simulink subsystem "Compute_LVLH_State"  (R2023a)
settings: Solver=VariableStepAuto  StartTime=0.0  StopTime=10.0  RelTol=1e-3
settings Model: Creator=Andy  LastModifiedBy=Andy

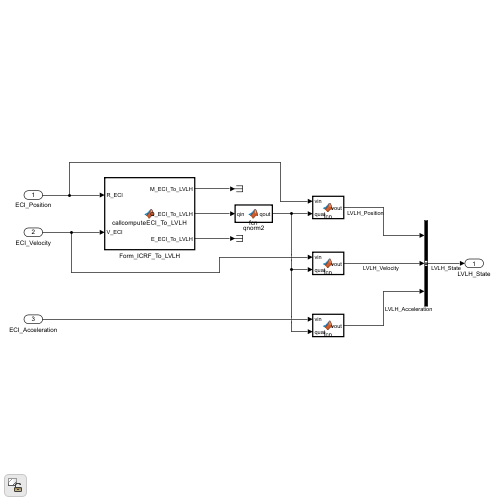
[thumbnail: Simulink's stored preview of the top-level diagram]
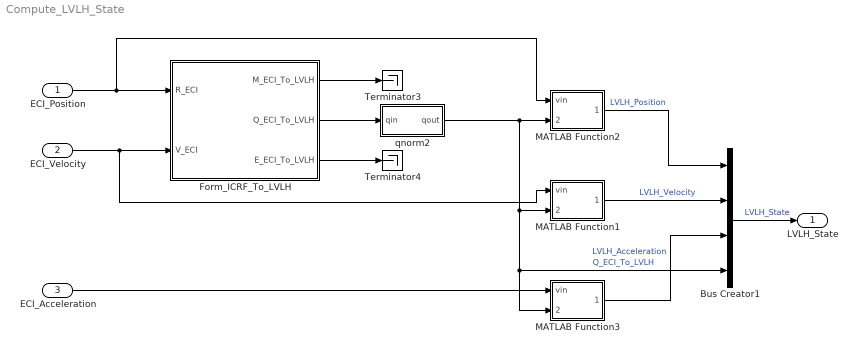
== system Compute_LVLH_State ==
  ECI_Position : Inport
  ECI_Velocity : Inport  Port=2
  ECI_Acceleration : Inport  Port=3
  Bus Creator1 : BusCreator  Inputs=4
  Form_ICRF_To_LVLH : MATLAB Function  TreatAsAtomicUnit=on
  MATLAB Function1 : MATLAB Function  TreatAsAtomicUnit=on
  MATLAB Function2 : MATLAB Function  TreatAsAtomicUnit=on
  MATLAB Function3 : MATLAB Function  TreatAsAtomicUnit=on
  Terminator3 : Terminator
  Terminator4 : Terminator
  qnorm2 : MATLAB Function  TreatAsAtomicUnit=on
  LVLH_State : Outport
  wires:
  Bus Creator1/1 -> LVLH_State/1  "LVLH_State"
  ECI_Acceleration/1 -> MATLAB Function3/1(vin)
  MATLAB Function1/1(vout) -> Bus Creator1/2  "LVLH_Velocity"
  Form_ICRF_To_LVLH/1(M_ECI_To_LVLH) -> Terminator3/1
  ECI_Position/1 -> Form_ICRF_To_LVLH/1(R_ECI), MATLAB Function2/1(vin)
  qnorm2/1(qout) -> MATLAB Function2/2(quat), MATLAB Function3/2(quat), Bus Creator1/4, MATLAB Function1/2(quat)  "Q_ECI_To_LVLH"
  MATLAB Function2/1(vout) -> Bus Creator1/1  "LVLH_Position"
  Form_ICRF_To_LVLH/3(E_ECI_To_LVLH) -> Terminator4/1
  Form_ICRF_To_LVLH/2(Q_ECI_To_LVLH) -> qnorm2/1(qin)
  ECI_Velocity/1 -> Form_ICRF_To_LVLH/2(V_ECI), MATLAB Function1/1(vin)
  MATLAB Function3/1(vout) -> Bus Creator1/3  "LVLH_Acceleration"

== matlab function Compute_LVLH_State/Form_ICRF_To_LVLH ==
  data: R_ECI input; M_ECI_To_LVLH output; Q_ECI_To_LVLH output; V_ECI input; E_ECI_To_LVLH output
function [M_ECI_To_LVLH,Q_ECI_To_LVLH,E_ECI_To_LVLH] = callcomputeECI_To_LVLH(R_ECI,V_ECI)


[M_ECI_To_LVLH,Q_ECI_To_LVLH,E_ECI_To_LVLH] = computeECI_To_LVLH(R_ECI,V_ECI);

== matlab function Compute_LVLH_State/MATLAB Function1 ==
  data: vin input; vout output; quat input
function vout = fcn(vin,quat)

vout = quatrotate(vin,quat);

== matlab function Compute_LVLH_State/MATLAB Function2 ==
  data: vin input; vout output; quat input
function vout = fcn(vin,quat)

vout = quatrotate(vin,quat);

== matlab function Compute_LVLH_State/MATLAB Function3 ==
  data: vin input; vout output; quat input
function vout = fcn(vin,quat)

vout = quatrotate(vin,quat);

== matlab function Compute_LVLH_State/qnorm2 ==
  data: qin input; qout output
function qout = fcn(qin)

qout = quatnorm(qin);
